simulink model "sampleModel167"  (R2021b)
settings: Solver=VariableStepAuto  StartTime=0.0  StopTime=10.0  RelTol=1e-3
undefined symbols (not defined in the file or in its folder): DiscIntNeverNeededParam
libraries: simulink x17, slpidlib x3, simulink_need_slupdate x2
settings Model: Creator=user  LastModifiedBy=user

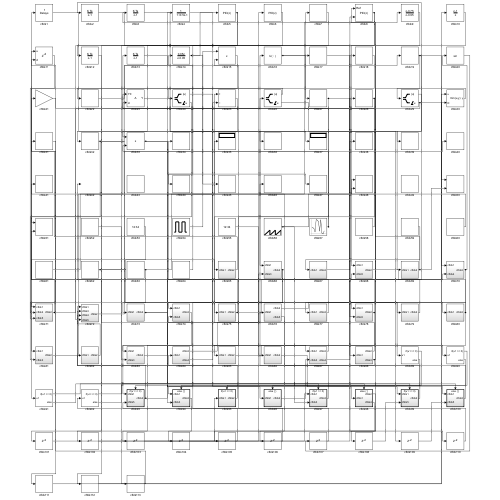
[thumbnail: Simulink's stored preview of the top-level diagram]
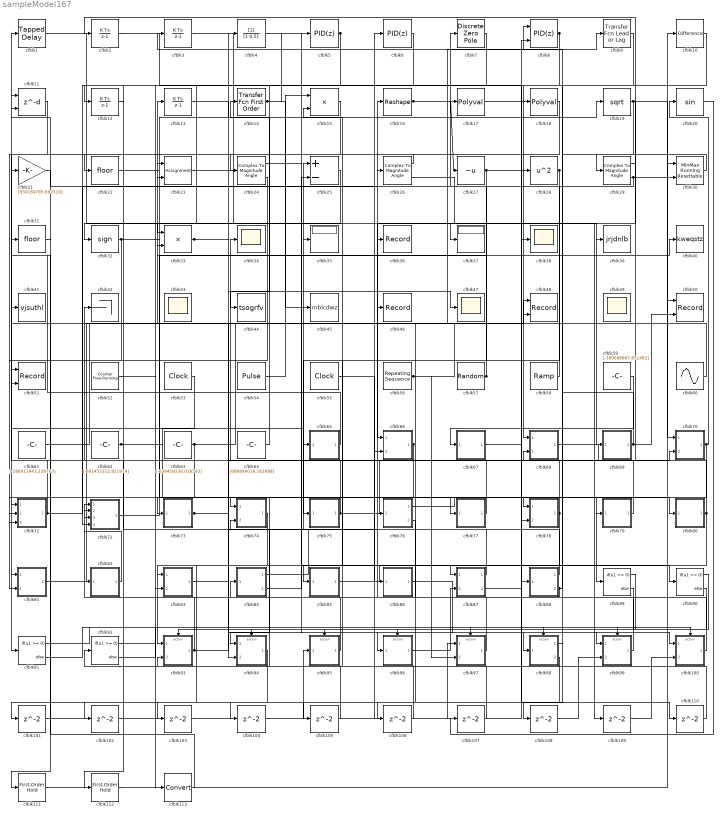
== system sampleModel167 ==
  cfblk1 : simulink/Discrete/Tapped Delay  vinit=0.0  samptime=-1  NumDelays=1  DelayOrder=Oldest  includeCurrent=off
  cfblk10 : simulink/Discrete/Difference  ICPrevInput=0.0  OutMin=[]  OutMax=[]  OutDataTypeStr=Inherit: Inherit via back propagation  OutDataType=fixdt(1, 16)  OutScaling=2^-10  DoSatur=off
  cfblk100 : Subsystem  TreatAsAtomicUnit=on
  cfblk{101..110} (10 alike) : Delay  SampleTime=1
  cfblk11 : Delay  DelayLengthSource=Input port  SampleTime=1
      settings: InputPortMap=u0,p1
  cfblk111 : simulink_need_slupdate/First-Order Hold  DisableCoverage=on  Ts=1
      settings: SourceProductBaseCode=SL
  cfblk112 : simulink_need_slupdate/First-Order Hold  DisableCoverage=on  Ts=1
      settings: SourceProductBaseCode=SL
  cfblk113 : DataTypeConversion
  cfblk{2..3,12..13} (4 alike) : DiscreteIntegrator  ICPrevOutput=DiscIntNeverNeededParam  ICPrevScaledInput=DiscIntNeverNeededParam
  cfblk14 : simulink/Discrete/Transfer Fcn First Order  PoleZ=0.95  ICPrevOutput=0.0  DoSatur=off
  cfblk15 : Product  Inputs=**
  cfblk16 : Reshape
  cfblk17 : Polyval  Coefs=[ +2.081618890e-019, -1.441693666e-014, +4.719686976e-010, -8.536869453e-006, +1.621573104e-001, -8.087801117e+001 ]
  cfblk18 : Polyval  Coefs=[ +2.081618890e-019, -1.441693666e-014, +4.719686976e-010, -8.536869453e-006, +1.621573104e-001, -8.087801117e+001 ]
  cfblk19 : Sqrt  SaturateOnIntegerOverflow=on
  cfblk20 : Trigonometry
  cfblk21 : Gain  Gain=[950169785.692510]
  cfblk22 : Rounding
  cfblk23 : Assignment  DiagnosticForDimensions=Warning  IndexOptions=Index vector (dialog)  Indices=1  OutputSizes=1
  cfblk24 : ComplexToMagnitudeAngle
  cfblk25 : Sum  Inputs=+-
  cfblk26 : ComplexToMagnitudeAngle
  cfblk27 : UnaryMinus
  cfblk28 : Math  Operator=square  SaturateOnIntegerOverflow=on
  cfblk29 : ComplexToMagnitudeAngle
  cfblk30 : simulink/Math Operations/MinMax Running Resettable  Function=min  vinit=0.0
  cfblk31 : Rounding
  cfblk32 : Signum
  cfblk33 : Product  Inputs=**
  cfblk{34,38,43,47,49} (5 alike) : Scope
      cfblk43 settings: Floating=on
      cfblk49 settings: Floating=on
  cfblk35 : Display
  cfblk36 : Record  FileSettingsInternal="{\"entries\":[{\"content\":{\"excelSettings\":{\"content\":{},\"type\":\"Streamout.ExcelSettings\"}},\"type\":\"Streamout.FileSettingStorage\",\"uuid\":\"ec53506d-30ea-4261-b9a0-b75c484f34c6\"}],\"packageUris\":[\"http://schema.mathworks.com/mf0/streamout_blocks/R2020a\"],\"version\":\"1.0\"}"  SignalsInternal="{\"entries\":[{\"content\":{\"signals\":[{\"content\":{\"blockPath\":[\"sampleModel167/cfblk36\"],\"channel\":[],\"dimensions\":[1],\"domain\":\"sampleModel167/cfblk36\",\"lineColor\":\"#0072bd\",\"plots\":[1],\"port\":1,\"sid\":[\"\"],\"signalID\":6249,\"signalName\":\"cfblk29:1\"},\"type\":\"RecordBlkView.Signal\",\"uuid\":\"139c6468-dbd3-450a-91ea-6cefff8656e1\"}]},\"type\":\"RecordBlkView.InputSignals\",\"uuid\":\"052d45fd-bfd9-46ee-adba-506bddab66a6\"}],\"packageUris\":[\"http://schema.mathworks.com/mf0/streamout_blocks/R2020a\"],\"version\":\"1.0\"}"  VisualizationBindings="{\"sparklinesplugin\":{\"info\":[{\"bindingParametersList\":[],\"subplotID\":1}]}}"
  cfblk37 : Display
  cfblk39 : ToWorkspace  VariableName=jrjdnlb  SaveFormat=Timeseries  SampleTime=-1
  cfblk4 : DiscreteFilter  SampleTime=1
  cfblk40 : ToWorkspace  VariableName=kweqstz  SaveFormat=Timeseries  SampleTime=-1
  cfblk41 : ToWorkspace  VariableName=vjsuthl  SaveFormat=Timeseries  SampleTime=-1
  cfblk42 : Terminator
  cfblk44 : ToWorkspace  VariableName=tsogrfv  SaveFormat=Timeseries  SampleTime=-1
  cfblk45 : ToWorkspace  VariableName=mblcdwz  SaveFormat=Timeseries  SampleTime=-1
  cfblk46 : Record  FileSettingsInternal="{\"entries\":[{\"content\":{\"excelSettings\":{\"content\":{},\"type\":\"Streamout.ExcelSettings\"}},\"type\":\"Streamout.FileSettingStorage\",\"uuid\":\"da6e1204-091f-4c4c-badc-bc2d25b8ce37\"}],\"packageUris\":[\"http://schema.mathworks.com/mf0/streamout_blocks/R2020a\"],\"version\":\"1.0\"}"  SignalsInternal="{\"entries\":[{\"content\":{\"signals\":[{\"content\":{\"blockPath\":[\"sampleModel167/cfblk46\"],\"channel\":[],\"dimensions\":[1],\"domain\":\"sampleModel167/cfblk46\",\"lineColor\":\"#d95319\",\"plots\":[1],\"port\":1,\"sid\":[\"\"],\"signalID\":6253,\"signalName\":\"cfblk100\"},\"type\":\"RecordBlkView.Signal\",\"uuid\":\"8a354596-a8b4-422e-ad70-63d130796eff\"}]},\"type\":\"RecordBlkView.InputSignals\",\"uuid\":\"d4f8df1c-8773-4cbd-9373-b1e680f83dd1\"}],\"packageUris\":[\"http://schema.mathworks.com/mf0/streamout_blocks/R2020a\"],\"version\":\"1.0\"}"  VisualizationBindings="{\"sparklinesplugin\":{\"info\":[{\"bindingParametersList\":[],\"subplotID\":1}]}}"
  cfblk48 : Record  FileSettingsInternal="{\"entries\":[{\"content\":{\"excelSettings\":{\"content\":{},\"type\":\"Streamout.ExcelSettings\"}},\"type\":\"Streamout.FileSettingStorage\",\"uuid\":\"2d2570bb-5f7a-4484-a74c-e022182345ca\"}],\"packageUris\":[\"http://schema.mathworks.com/mf0/streamout_blocks/R2020a\"],\"version\":\"1.0\"}"  Layout=[1 1]  SignalsInternal="{\"entries\":[{\"content\":{\"signals\":[{\"content\":{\"blockPath\":[\"sampleModel167/cfblk48\"],\"channel\":[],\"dimensions\":[1],\"domain\":\"sampleModel167/cfblk48\",\"lineColor\":\"#a2142f\",\"plots\":[1],\"port\":1,\"sid\":[\"\"],\"signalID\":6257,\"signalName\":\"cfblk80\"},\"type\":\"RecordBlkView.Signal\",\"uuid\":\"0f420bdd-d17e-44a9-89a2-4def85ddcdf1\"},{\"content\":{\"blockPath\":[\"sampleModel167/cfblk48\"],\"channel\":[],\"dimensions\":[1],\"domain\":\"sampleModel167/cfblk48\",\"lineColor\":\"#139fff\",\"plots\":[1],\"port\":2,\"sid\":[\"\"],\"signalID\":6261,\"signalName\":\"cfblk73\"},\"type\":\"RecordBlkView.Signal\",\"uuid\":\"37ea3ef6-358e-4351-b671-b7f0163bc937\"}]},\"type\":\"RecordBlkView.InputSignals\",\"uuid\":\"119d5875-aaf2-4c77-af19-f5638ded1561\"}],\"packageUris\":[\"http://schema.mathworks.com/mf0/streamout_blocks/R2020a\"],\"version\":\"1.0\"}"  VisualizationBindings="{\"xyplotplugin\":{\"info\":[{\"series\":[{\"bindingParametersList\":[{\"parameter\":\"X-Axis\",\"signalID\":6257,\"signalName\":\"cfblk80\"},{\"parameter\":\"Y-Axis\",\"signalID\":6261,\"signalName\":\"cfblk73\"}],\"seriesID\":53970}],\"subplotID\":1}]}}"  CompatibilityTag=XY
  cfblk5 : slpidlib/PID Controller  Controller=PID  Form=Parallel  TimeDomain=Discrete-time  UseExternalTs=off  SampleTime=1  IntegratorMethod=Forward Euler  FilterMethod=Forward Euler  ControllerParametersSource=internal  P=1  I=1  D=0  UseFilter=on  N=100  TunerSelectOption=Transfer Function Based (PID Tuner App)  InitialConditionSource=internal  InitialConditionForIntegrator=0  InitialConditionForFilter=0  DifferentiatorICPrevScaledInput=0  ExternalReset=none  TrackingMode=off  Kt=1  LimitOutput=off  SatLimitsSource=internal  UpperSaturationLimit=inf  LowerSaturationLimit=-inf  LinearizeAsGain=off  AntiWindupMode=none  Kb=1  POutMin=[]  POutMax=[]  IOutMin=[]  IOutMax=[]  DOutMin=[]  DOutMax=[]  NOutMin=[]  NOutMax=[]  SumOutMin=[]  SumOutMax=[]  SaturationOutMin=[]  SaturationOutMax=[]  PParamMin=[]  PParamMax=[]  IParamMin=[]  IParamMax=[]  DParamMin=[]  DParamMax=[]  NParamMin=[]  NParamMax=[]  KbParamMin=[]  KbParamMax=[]  KtParamMin=[]  KtParamMax=[]  KbOutMin=[]  KbOutMax=[]  KtOutMin=[]  KtOutMax=[]  IntegratorOutMin=[]  IntegratorOutMax=[]  FilterOutMin=[]  FilterOutMax=[]  SumI1OutMin=[]  SumI1OutMax=[]  SumI2OutMin=[]  SumI2OutMax=[]  SumI3OutMin=[]  SumI3OutMax=[]  SumI4OutMin=[]  SumI4OutMax=[]  SumDOutMin=[]  SumDOutMax=[]  DifferentiatorOutMin=[]  DifferentiatorOutMax=[]  FilterDiffOutCoefMin=[]  FilterDiffOutCoefMax=[]  ReciprocalOutMin=[]  ReciprocalOutMax=[]  SumDenOutMin=[]  SumDenOutMax=[]  SumNumOutMin=[]  SumNumOutMax=[]  DivideOutMin=[]  DivideOutMax=[]  UdiffTsProdOutMin=[]  UdiffTsProdOutMax=[]  NTsProdOutMin=[]  NTsProdOutMax=[]  UintegralTsProdOutMin=[]  UintegralTsProdOutMax=[]  UngainTsProdOutMin=[]  UngainTsProdOutMax=[]  IntegratorContinuousStateAttributes=''  IntegratorStateMustResolveToSignalObject=off  IntegratorRTWStateStorageClass=Auto  FilterContinuousStateAttributes=''  FilterStateMustResolveToSignalObject=off  FilterRTWStateStorageClass=Auto  ParallelPVariant=InternalParameters  IdealPVariant=Disabled  IVariant=InternalParameters  DVariant=InternalParameters  IntegratorVariant=Discrete  SatVariant=Disabled  AWVariant=Passthrough  PCopyVariant=Disabled  TRVariant=Disabled  FdbkBlocksVariant=Forward  IdealPFdbkVariant=Disabled  SatFdbkVariant=Disabled  DerivativeFilterVariant=ForwardEulerFilter  NVariant=InternalParameters  NCopyVariant=Disabled  FilterICVariant=InternalICsFilter  IntegratorICVariant=InternalICs  ExternalResetVariant=Disabled  TRSumVariant=Passthrough  SumFdbkVariant=Disabled  SumVariant=Sum_PID  TsampFilterVariant=InternalTs  TsampNgainVariant=Passthrough  TsampIntegralVariant=Passthrough  ExternalSaturationOutDataTypeStr=Inherit: Same as second input
  cfblk50 : Record  FileSettingsInternal="{\"entries\":[{\"content\":{\"excelSettings\":{\"content\":{},\"type\":\"Streamout.ExcelSettings\"}},\"type\":\"Streamout.FileSettingStorage\",\"uuid\":\"40a77355-b6b9-4623-865c-1ca23200a22d\"}],\"packageUris\":[\"http://schema.mathworks.com/mf0/streamout_blocks/R2020a\"],\"version\":\"1.0\"}"  Layout=[1 1]  SignalsInternal="{\"entries\":[{\"content\":{\"signals\":[{\"content\":{\"blockPath\":[\"sampleModel167/cfblk50\"],\"channel\":[],\"dimensions\":[1],\"domain\":\"sampleModel167/cfblk50\",\"lineColor\":\"#a2142f\",\"plots\":[1],\"port\":1,\"sid\":[\"\"],\"signalID\":6265,\"signalName\":\"cfblk29:2\"},\"type\":\"RecordBlkView.Signal\",\"uuid\":\"cc7a997b-e63d-444a-905f-d59d5b2896fd\"},{\"content\":{\"blockPath\":[\"sampleModel167/cfblk50\"],\"channel\":[],\"dimensions\":[1],\"domain\":\"sampleModel167/cfblk50\",\"lineColor\":\"#139fff\",\"plots\":[1],\"port\":2,\"sid\":[\"\"],\"signalID\":6269,\"signalName\":\"cfblk69\"},\"type\":\"RecordBlkView.Signal\",\"uuid\":\"124d10ed-abfe-4519-b392-b2a6d6e38794\"}]},\"type\":\"RecordBlkView.InputSignals\",\"uuid\":\"67c040a3-84bd-4415-84fd-296e2aa30a4d\"}],\"packageUris\":[\"http://schema.mathworks.com/mf0/streamout_blocks/R2020a\"],\"version\":\"1.0\"}"  VisualizationBindings="{\"xyplotplugin\":{\"info\":[{\"series\":[{\"bindingParametersList\":[{\"parameter\":\"X-Axis\",\"signalID\":6265,\"signalName\":\"cfblk29:2\"},{\"parameter\":\"Y-Axis\",\"signalID\":6269,\"signalName\":\"cfblk69\"}],\"seriesID\":27313}],\"subplotID\":1}]}}"  CompatibilityTag=XY
  cfblk51 : Record  FileSettingsInternal="{\"entries\":[{\"content\":{\"excelSettings\":{\"content\":{},\"type\":\"Streamout.ExcelSettings\"}},\"type\":\"Streamout.FileSettingStorage\",\"uuid\":\"e3204bcf-3174-4af1-beb2-6810d04cfba5\"}],\"packageUris\":[\"http://schema.mathworks.com/mf0/streamout_blocks/R2020a\"],\"version\":\"1.0\"}"  Layout=[1 1]  SignalsInternal="{\"entries\":[{\"content\":{\"signals\":[{\"content\":{\"blockPath\":[\"sampleModel167/cfblk51\"],\"channel\":[],\"dimensions\":[1],\"domain\":\"sampleModel167/cfblk51\",\"lineColor\":\"#a2142f\",\"plots\":[1],\"port\":1,\"sid\":[\"\"],\"signalID\":6273,\"signalName\":\"cfblk24:2\"},\"type\":\"RecordBlkView.Signal\",\"uuid\":\"6600f92a-317f-4508-8dc5-cdf654def4ef\"},{\"content\":{\"blockPath\":[\"sampleModel167/cfblk51\"],\"channel\":[],\"dimensions\":[1],\"domain\":\"sampleModel167/cfblk51\",\"lineColor\":\"#139fff\",\"plots\":[1],\"port\":2,\"sid\":[\"\"],\"signalID\":6277,\"signalName\":\"cfblk71\"},\"type\":\"RecordBlkView.Signal\",\"uuid\":\"6d6ba4b2-e462-4f03-bdb0-15236c8ce066\"}]},\"type\":\"RecordBlkView.InputSignals\",\"uuid\":\"fb1d1275-7641-4af6-b3e0-80677102a4a7\"}],\"packageUris\":[\"http://schema.mathworks.com/mf0/streamout_blocks/R2020a\"],\"version\":\"1.0\"}"  VisualizationBindings="{\"xyplotplugin\":{\"info\":[{\"series\":[{\"bindingParametersList\":[{\"parameter\":\"X-Axis\",\"signalID\":6273,\"signalName\":\"cfblk24:2\"},{\"parameter\":\"Y-Axis\",\"signalID\":6277,\"signalName\":\"cfblk71\"}],\"seriesID\":11353}],\"subplotID\":1}]}}"  CompatibilityTag=XY
  cfblk52 : simulink/Sources/Counter Free-Running  NumBits=[41.000000]  tsamp=-1
  cfblk53 : DigitalClock
  cfblk54 : DiscretePulseGenerator  PulseType=Time based  Amplitude=[534137876.527184]  Period=[54976083.843764]  PulseWidth=5  PhaseDelay=[8.000000]
  cfblk55 : DigitalClock
  cfblk56 : simulink/Sources/Repeating Sequence  rep_seq_t=[0 2]  rep_seq_y=[-841539136.031872, -579381442.323745]
  cfblk57 : RandomNumber  Mean=[-51850.961878]  Variance=[97939.194317]  Seed=[432152080.000000]  SampleTime=0.1
  cfblk58 : simulink/Sources/Ramp  slope=[-4478.791088]  start=[26.895940]  InitialOutput=[-682797.916035]
  cfblk59 : Constant  Value=[-369688867.851482]  SampleTime=1
  cfblk6 : slpidlib/PID Controller  Controller=PID  Form=Parallel  TimeDomain=Discrete-time  UseExternalTs=off  SampleTime=1  IntegratorMethod=Forward Euler  FilterMethod=Forward Euler  ControllerParametersSource=internal  P=1  I=1  D=0  UseFilter=on  N=100  TunerSelectOption=Transfer Function Based (PID Tuner App)  InitialConditionSource=internal  InitialConditionForIntegrator=0  InitialConditionForFilter=0  DifferentiatorICPrevScaledInput=0  ExternalReset=none  TrackingMode=off  Kt=1  LimitOutput=off  SatLimitsSource=internal  UpperSaturationLimit=inf  LowerSaturationLimit=-inf  LinearizeAsGain=off  AntiWindupMode=none  Kb=1  POutMin=[]  POutMax=[]  IOutMin=[]  IOutMax=[]  DOutMin=[]  DOutMax=[]  NOutMin=[]  NOutMax=[]  SumOutMin=[]  SumOutMax=[]  SaturationOutMin=[]  SaturationOutMax=[]  PParamMin=[]  PParamMax=[]  IParamMin=[]  IParamMax=[]  DParamMin=[]  DParamMax=[]  NParamMin=[]  NParamMax=[]  KbParamMin=[]  KbParamMax=[]  KtParamMin=[]  KtParamMax=[]  KbOutMin=[]  KbOutMax=[]  KtOutMin=[]  KtOutMax=[]  IntegratorOutMin=[]  IntegratorOutMax=[]  FilterOutMin=[]  FilterOutMax=[]  SumI1OutMin=[]  SumI1OutMax=[]  SumI2OutMin=[]  SumI2OutMax=[]  SumI3OutMin=[]  SumI3OutMax=[]  SumI4OutMin=[]  SumI4OutMax=[]  SumDOutMin=[]  SumDOutMax=[]  DifferentiatorOutMin=[]  DifferentiatorOutMax=[]  FilterDiffOutCoefMin=[]  FilterDiffOutCoefMax=[]  ReciprocalOutMin=[]  ReciprocalOutMax=[]  SumDenOutMin=[]  SumDenOutMax=[]  SumNumOutMin=[]  SumNumOutMax=[]  DivideOutMin=[]  DivideOutMax=[]  UdiffTsProdOutMin=[]  UdiffTsProdOutMax=[]  NTsProdOutMin=[]  NTsProdOutMax=[]  UintegralTsProdOutMin=[]  UintegralTsProdOutMax=[]  UngainTsProdOutMin=[]  UngainTsProdOutMax=[]  IntegratorContinuousStateAttributes=''  IntegratorStateMustResolveToSignalObject=off  IntegratorRTWStateStorageClass=Auto  FilterContinuousStateAttributes=''  FilterStateMustResolveToSignalObject=off  FilterRTWStateStorageClass=Auto  ParallelPVariant=InternalParameters  IdealPVariant=Disabled  IVariant=InternalParameters  DVariant=InternalParameters  IntegratorVariant=Discrete  SatVariant=Disabled  AWVariant=Passthrough  PCopyVariant=Disabled  TRVariant=Disabled  FdbkBlocksVariant=Forward  IdealPFdbkVariant=Disabled  SatFdbkVariant=Disabled  DerivativeFilterVariant=ForwardEulerFilter  NVariant=InternalParameters  NCopyVariant=Disabled  FilterICVariant=InternalICsFilter  IntegratorICVariant=InternalICs  ExternalResetVariant=Disabled  TRSumVariant=Passthrough  SumFdbkVariant=Disabled  SumVariant=Sum_PID  TsampFilterVariant=InternalTs  TsampNgainVariant=Passthrough  TsampIntegralVariant=Passthrough  ExternalSaturationOutDataTypeStr=Inherit: Same as second input
  cfblk60 : Sin  Amplitude=[-473951708.743377]  Bias=[-825559147.344328]  SampleTime=0
  cfblk61 : Constant  Value=[-188911943.228703]  SampleTime=1
  cfblk62 : Constant  Value=[-601452312.821979]  SampleTime=1
  cfblk63 : Constant  Value=[-638459236.016593]  SampleTime=1
  cfblk64 : Constant  Value=[686890016.162688]  SampleTime=1
  cfblk65 : Subsystem
  cfblk66 : Subsystem
  cfblk67 : Subsystem
  cfblk68 : Subsystem
  cfblk69 : Subsystem
  cfblk7 : DiscreteZeroPole  Poles=[0 0.5]  Gain=1
  cfblk70 : Subsystem
  cfblk71 : Subsystem
  cfblk72 : Subsystem
  cfblk73 : Subsystem
  cfblk74 : Subsystem
  cfblk75 : Subsystem
  cfblk76 : Subsystem
  cfblk77 : Subsystem
  cfblk78 : Subsystem
  cfblk79 : Subsystem
  cfblk8 : slpidlib/PID Controller (2DOF)  Controller=PID  Form=Parallel  TimeDomain=Discrete-time  UseExternalTs=off  SampleTime=1  IntegratorMethod=Forward Euler  FilterMethod=Forward Euler  ControllerParametersSource=internal  P=1  I=1  D=0  UseFilter=on  N=100  b=1  c=1  TunerSelectOption=Transfer Function Based (PID Tuner App)  InitialConditionSource=internal  InitialConditionForIntegrator=0  InitialConditionForFilter=0  DifferentiatorICPrevScaledInput=0  ExternalReset=none  TrackingMode=off  Kt=1  LimitOutput=off  SatLimitsSource=internal  UpperSaturationLimit=inf  LowerSaturationLimit=-inf  LinearizeAsGain=off  AntiWindupMode=none  Kb=1  POutMin=[]  POutMax=[]  IOutMin=[]  IOutMax=[]  DOutMin=[]  DOutMax=[]  NOutMin=[]  NOutMax=[]  bOutMin=[]  bOutMax=[]  cOutMin=[]  cOutMax=[]  SumOutMin=[]  SumOutMax=[]  SaturationOutMin=[]  SaturationOutMax=[]  PParamMin=[]  PParamMax=[]  IParamMin=[]  IParamMax=[]  DParamMin=[]  DParamMax=[]  NParamMin=[]  NParamMax=[]  bParamMin=[]  bParamMax=[]  cParamMin=[]  cParamMax=[]  KbParamMin=[]  KbParamMax=[]  KtParamMin=[]  KtParamMax=[]  KbOutMin=[]  KbOutMax=[]  KtOutMin=[]  KtOutMax=[]  IntegratorOutMin=[]  IntegratorOutMax=[]  FilterOutMin=[]  FilterOutMax=[]  SumI1OutMin=[]  SumI1OutMax=[]  SumI2OutMin=[]  SumI2OutMax=[]  SumI3OutMin=[]  SumI3OutMax=[]  SumI4OutMin=[]  SumI4OutMax=[]  SumDOutMin=[]  SumDOutMax=[]  Sum1OutMin=[]  Sum1OutMax=[]  Sum2OutMin=[]  Sum2OutMax=[]  Sum3OutMin=[]  Sum3OutMax=[]  DifferentiatorOutMin=[]  DifferentiatorOutMax=[]  FilterDiffOutCoefMin=[]  FilterDiffOutCoefMax=[]  ReciprocalOutMin=[]  ReciprocalOutMax=[]  SumDenOutMin=[]  SumDenOutMax=[]  SumNumOutMin=[]  SumNumOutMax=[]  DivideOutMin=[]  DivideOutMax=[]  UdiffTsProdOutMin=[]  UdiffTsProdOutMax=[]  NTsProdOutMin=[]  NTsProdOutMax=[]  UintegralTsProdOutMin=[]  UintegralTsProdOutMax=[]  UngainTsProdOutMin=[]  UngainTsProdOutMax=[]  IntegratorContinuousStateAttributes=''  IntegratorStateMustResolveToSignalObject=off  IntegratorRTWStateStorageClass=Auto  FilterContinuousStateAttributes=''  FilterStateMustResolveToSignalObject=off  FilterRTWStateStorageClass=Auto  ParallelPVariant=InternalParameters  IdealPVariant=Disabled  IVariant=InternalParameters  DVariant=InternalParameters  bVariant=InternalParameters  cVariant=InternalParameters  IntegratorVariant=Discrete  SatVariant=Disabled  AWVariant=Passthrough  PCopyVariant=Disabled  TRVariant=Disabled  FdbkBlocksVariant=Forward  IdealPFdbkVariant=Disabled  SatFdbkVariant=Disabled  DerivativeFilterVariant=ForwardEulerFilter  NVariant=InternalParameters  NCopyVariant=Disabled  FilterICVariant=InternalICsFilter  IntegratorICVariant=InternalICs  ExternalResetVariant=Disabled  TRSumVariant=Passthrough  SumFdbkVariant=Disabled  SumVariant=Sum_PID  TsampFilterVariant=InternalTs  TsampNgainVariant=Passthrough  TsampIntegralVariant=Passthrough  ExternalSaturationOutDataTypeStr=Inherit: Same as second input
      settings: SourceProductBaseCode=SL
  cfblk80 : Subsystem
  cfblk81 : Subsystem
  cfblk82 : Subsystem
  cfblk83 : Subsystem
  cfblk84 : Subsystem
  cfblk85 : Subsystem
  cfblk86 : Subsystem
  cfblk87 : Subsystem
  cfblk88 : Subsystem
  cfblk{89..92} (4 alike) : If  IfExpression=u1 >= 0  SampleTime=1
  cfblk9 : simulink/Discrete/Transfer Fcn Lead or Lag  PoleZ=0.95  ZeroZ=0.75  ICPrevOutput=0.0  ICPrevInput=0.0  DoSatur=off
      settings: SourceProductBaseCode=SL
  cfblk93 : Subsystem  TreatAsAtomicUnit=on
  cfblk94 : Subsystem  TreatAsAtomicUnit=on
  cfblk95 : Subsystem  TreatAsAtomicUnit=on
  cfblk96 : Subsystem  TreatAsAtomicUnit=on
  cfblk97 : Subsystem  TreatAsAtomicUnit=on
  cfblk98 : Subsystem  TreatAsAtomicUnit=on
  cfblk99 : Subsystem  TreatAsAtomicUnit=on
  wires:
  cfblk54/1 -> cfblk15/1
  cfblk25/1 -> cfblk32/1
  cfblk62/1 -> cfblk89/1, cfblk65/1(cfblk1)
  cfblk58/1 -> cfblk7/1
  cfblk16/1 -> cfblk27/1, cfblk9/1
  cfblk70/1(cfblk2) -> cfblk74/1(cfblk1), cfblk20/1
  cfblk88/1(cfblk2) -> cfblk1/1
  cfblk97/1(cfblk2) -> cfblk16/1
  cfblk69/1(cfblk2) -> cfblk8/1, cfblk50/2
  cfblk1/1 -> cfblk66/1(cfblk1)
  cfblk75/1(cfblk2) -> cfblk42/1, cfblk10/1
  cfblk61/1 -> cfblk13/1
  cfblk68/1(cfblk2) -> cfblk2/1
  cfblk79/1(cfblk2) -> cfblk11/1
  cfblk66/1(cfblk2) -> cfblk94/1(cfblk1), cfblk73/1(cfblk1)
  cfblk81/1(cfblk2) -> cfblk17/1
  cfblk11/1 -> cfblk91/1
  cfblk60/1 -> cfblk41/1
  cfblk77/1(cfblk2) -> cfblk34/1
  cfblk32/1 -> cfblk80/1(cfblk1), cfblk19/1, cfblk71/2(cfblk4)
  cfblk65/1(cfblk2) -> cfblk21/1
  cfblk59/1 -> cfblk67/1(cfblk1)
  cfblk14/1 -> cfblk5/1, cfblk45/1
  cfblk10/1 -> cfblk68/1(cfblk1)
  cfblk53/1 -> cfblk81/1(cfblk1)
  cfblk4/1 -> cfblk96/1(cfblk1)
  cfblk3/1 -> cfblk37/1
  cfblk13/1 -> cfblk94/2(cfblk3)
  cfblk93/1(cfblk2) -> cfblk72/1(cfblk1), cfblk76/1(cfblk1)
  cfblk6/1 -> cfblk12/1
  cfblk76/1(cfblk2) -> cfblk79/1(cfblk1)
  cfblk100/1(cfblk2) -> cfblk46/1
  cfblk71/1(cfblk2) -> cfblk26/1, cfblk51/2
  cfblk63/1 -> cfblk25/1, cfblk71/3(cfblk5)
  cfblk67/1(cfblk2) -> cfblk38/1
  cfblk21/1 -> cfblk71/1(cfblk1)
  cfblk74/1(cfblk2) -> cfblk93/1(cfblk1)
  cfblk86/1(cfblk2) -> cfblk98/1(cfblk1)
  cfblk57/1 -> cfblk11/2, cfblk33/2
  cfblk80/1(cfblk2) -> cfblk83/1(cfblk1), cfblk77/1(cfblk1), cfblk48/1
  cfblk29/1 -> cfblk36/1
  cfblk9/1 -> cfblk78/1(cfblk1)
  cfblk72/1(cfblk2) -> cfblk40/1
  cfblk78/1(cfblk2) -> cfblk68/2(cfblk5), cfblk103/1
  cfblk33/1 -> cfblk47/1, cfblk99/1(cfblk1)
  cfblk5/1 -> cfblk44/1, cfblk33/1
  cfblk73/1(cfblk2) -> cfblk100/1(cfblk1), cfblk48/2
  cfblk87/1(cfblk2) -> cfblk35/1
  cfblk23/1 -> cfblk69/1(cfblk1)
  cfblk85/1(cfblk2) -> cfblk90/1
  cfblk27/1 -> cfblk78/2(cfblk5), cfblk85/1(cfblk1)
  cfblk95/1(cfblk2) -> cfblk72/2(cfblk3)
  cfblk56/1 -> cfblk28/1, cfblk97/2(cfblk3)
  cfblk19/1 -> cfblk70/1(cfblk1), cfblk39/1, cfblk108/1
  cfblk55/1 -> cfblk86/1(cfblk1)
  cfblk24/1 -> cfblk87/1(cfblk1)
  cfblk28/1 -> cfblk75/1(cfblk1), cfblk23/2
  cfblk64/1 -> cfblk14/1
  cfblk15/1 -> cfblk81/2(cfblk3)
  cfblk22/1 -> cfblk4/1
  cfblk84/1(cfblk2) -> cfblk6/1
  cfblk2/1 -> cfblk88/1(cfblk1)
  cfblk99/1(cfblk2) -> cfblk84/1(cfblk1)
  cfblk96/1(cfblk2) -> cfblk87/2(cfblk3)
  cfblk26/1 -> cfblk24/1
  cfblk83/1(cfblk2) -> cfblk70/2(cfblk4)
  cfblk24/2 -> cfblk51/1
  cfblk84/2(cfblk4) -> cfblk25/2
  cfblk87/2(cfblk4) -> cfblk18/1
  cfblk7/1 -> cfblk22/1
  cfblk88/2(cfblk3) -> cfblk82/1(cfblk1), cfblk3/1
  cfblk29/2 -> cfblk50/1, cfblk23/1
  cfblk30/1 -> cfblk29/1
  cfblk8/1 -> cfblk83/2(cfblk3), cfblk72/4(cfblk5)
  cfblk82/1(cfblk2) -> cfblk72/3(cfblk4)
  cfblk89/1 -> cfblk93/Action
  cfblk89/2 -> cfblk94/Action
  cfblk90/1 -> cfblk95/Action
  cfblk90/2 -> cfblk96/Action
  cfblk91/1 -> cfblk97/Action
  cfblk91/2 -> cfblk98/Action
  cfblk92/1 -> cfblk99/Action
  cfblk92/2 -> cfblk100/Action
  cfblk94/1(cfblk2) -> cfblk101/1
  cfblk101/1 -> cfblk66/2(cfblk3)
  cfblk18/1 -> cfblk102/1
  cfblk102/1 -> cfblk95/1(cfblk1)
  cfblk103/1 -> cfblk97/1(cfblk1)
  cfblk98/1(cfblk2) -> cfblk104/1
  cfblk104/1 -> cfblk8/2
  cfblk98/2(cfblk4) -> cfblk105/1
  cfblk105/1 -> cfblk93/2(cfblk5)
  cfblk76/2(cfblk5) -> cfblk106/1
  cfblk106/1 -> cfblk74/2(cfblk5)
  cfblk20/1 -> cfblk107/1
  cfblk107/1 -> cfblk92/1
  cfblk108/1 -> cfblk99/2(cfblk5)
  cfblk26/2 -> cfblk109/1
  cfblk109/1 -> cfblk100/2(cfblk5)
  cfblk17/1 -> cfblk110/1
  cfblk110/1 -> cfblk15/2
  cfblk31/1 -> cfblk111/1
  cfblk111/1 -> cfblk30/1
  cfblk12/1 -> cfblk112/1
  cfblk112/1 -> cfblk30/2
  cfblk52/1 -> cfblk113/1
  cfblk113/1 -> cfblk31/1

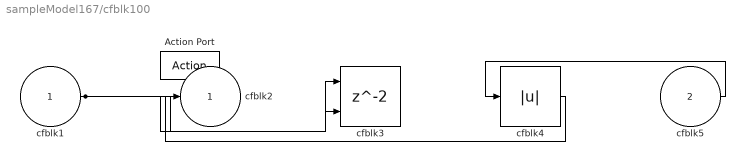
== system sampleModel167/cfblk100 ==
  cfblk1 : Inport
  cfblk5 : Inport  Port=2
  Action Port : ActionPort  ActionPortLabel=else
  cfblk3 : Delay  ShowEnablePort=on
      settings: InputPortMap=u0,e6
  cfblk4 : Abs
  cfblk2 : Outport
  wires:
  cfblk5/1 -> cfblk4/1
  cfblk1/1 -> cfblk3/1, cfblk3/2
  cfblk4/1 -> cfblk2/1

== system sampleModel167/cfblk65 ==
  cfblk1 : Inport
  cfblk3 : Sin  TimeSource=Use external signal  SampleTime=0
  cfblk4 : Constant  Value=[688240254.247042]  SampleTime=1
  cfblk2 : Outport
  wires:
  cfblk1/1 -> cfblk2/1
  cfblk4/1 -> cfblk3/1

== system sampleModel167/cfblk66 ==
  cfblk1 : Inport
  cfblk3 : Inport  Port=2
  cfblk2 : Outport
  wires:
  cfblk1/1 -> cfblk2/1

== system sampleModel167/cfblk67 ==
  cfblk1 : Inport
  cfblk3 : Constant  Value=[170733425.297575]  SampleTime=1
  cfblk2 : Outport
  wires:
  cfblk3/1 -> cfblk2/1

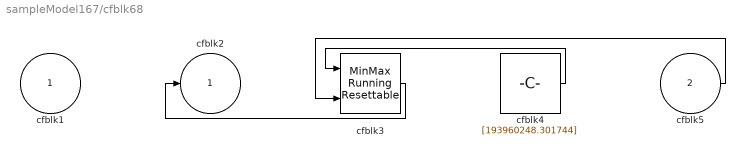
== system sampleModel167/cfblk68 ==
  cfblk1 : Inport
  cfblk5 : Inport  Port=2
  cfblk3 : simulink/Math Operations/MinMax Running Resettable  Function=min  vinit=0.0
  cfblk4 : Constant  Value=[193960248.301744]  SampleTime=1
  cfblk2 : Outport
  wires:
  cfblk4/1 -> cfblk3/1
  cfblk3/1 -> cfblk2/1
  cfblk5/1 -> cfblk3/2

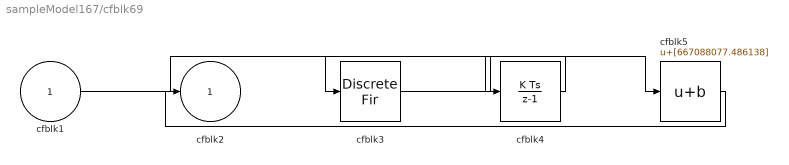
== system sampleModel167/cfblk69 ==
  cfblk1 : Inport
  cfblk3 : DiscreteFir  SampleTime=1
  cfblk4 : DiscreteIntegrator  ICPrevOutput=DiscIntNeverNeededParam  ICPrevScaledInput=DiscIntNeverNeededParam
  cfblk5 : Bias  Bias=[667088077.486138]
  cfblk2 : Outport
  wires:
  cfblk3/1 -> cfblk5/1
  cfblk1/1 -> cfblk4/1
  cfblk5/1 -> cfblk2/1
  cfblk4/1 -> cfblk3/1

== system sampleModel167/cfblk70 ==
  cfblk1 : Inport
  cfblk4 : Inport  Port=2
  cfblk3 : simulink/Discrete/Tapped Delay  vinit=0.0  samptime=-1  NumDelays=1  DelayOrder=Oldest  includeCurrent=off
  cfblk2 : Outport
  wires:
  cfblk1/1 -> cfblk2/1
  cfblk4/1 -> cfblk3/1

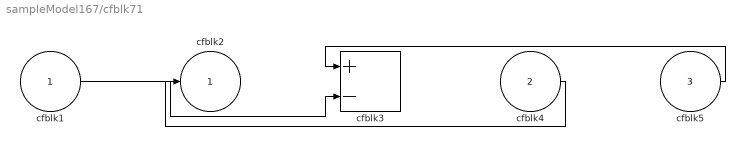
== system sampleModel167/cfblk71 ==
  cfblk1 : Inport
  cfblk4 : Inport  Port=2
  cfblk5 : Inport  Port=3
  cfblk3 : Sum  Inputs=+-
  cfblk2 : Outport
  wires:
  cfblk5/1 -> cfblk3/1
  cfblk1/1 -> cfblk3/2
  cfblk4/1 -> cfblk2/1

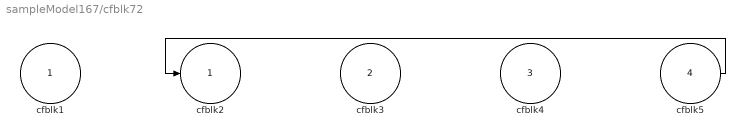
== system sampleModel167/cfblk72 ==
  cfblk1 : Inport
  cfblk3 : Inport  Port=2
  cfblk4 : Inport  Port=3
  cfblk5 : Inport  Port=4
  cfblk2 : Outport
  wires:
  cfblk5/1 -> cfblk2/1

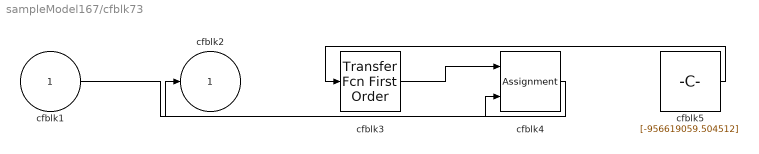
== system sampleModel167/cfblk73 ==
  cfblk1 : Inport
  cfblk3 : simulink/Discrete/Transfer Fcn First Order  PoleZ=0.95  ICPrevOutput=0.0  DoSatur=off
  cfblk4 : Assignment  DiagnosticForDimensions=Warning  IndexOptions=Index vector (dialog)  Indices=1  OutputSizes=1
  cfblk5 : Constant  Value=[-956619059.504512]  SampleTime=1
  cfblk2 : Outport
  wires:
  cfblk5/1 -> cfblk3/1
  cfblk3/1 -> cfblk4/1
  cfblk4/1 -> cfblk2/1
  cfblk1/1 -> cfblk4/2

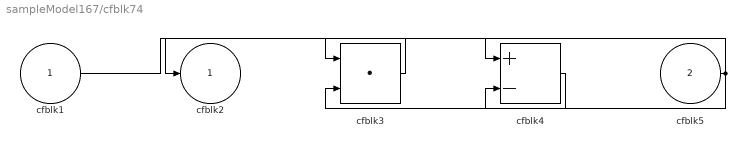
== system sampleModel167/cfblk74 ==
  cfblk1 : Inport
  cfblk5 : Inport  Port=2
  cfblk3 : DotProduct  InputSameDT=on  OutDataTypeStr=Inherit: Inherit via internal rule
  cfblk4 : Sum  Inputs=+-
  cfblk2 : Outport
  wires:
  cfblk5/1 -> cfblk3/1, cfblk4/2
  cfblk4/1 -> cfblk3/2
  cfblk3/1 -> cfblk2/1
  cfblk1/1 -> cfblk4/1

== system sampleModel167/cfblk75 ==
  cfblk1 : Inport
  cfblk3 : Trigonometry
  cfblk2 : Outport
  wires:
  cfblk3/1 -> cfblk2/1
  cfblk1/1 -> cfblk3/1

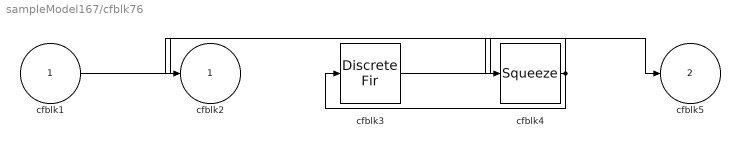
== system sampleModel167/cfblk76 ==
  cfblk1 : Inport
  cfblk3 : DiscreteFir  SampleTime=1
  cfblk4 : Squeeze
  cfblk2 : Outport
  cfblk5 : Outport  Port=2
  wires:
  cfblk3/1 -> cfblk5/1
  cfblk1/1 -> cfblk4/1
  cfblk4/1 -> cfblk3/1, cfblk2/1

== system sampleModel167/cfblk77 ==
  cfblk1 : Inport
  cfblk3 : DiscreteTransferFcn  SampleTime=1
  cfblk4 : Sum  Inputs=-+
  cfblk5 : simulink/Math Operations/Slider Gain  gain=1  low=0  high=2
  cfblk2 : Outport
  wires:
  cfblk1/1 -> cfblk3/1
  cfblk3/1 -> cfblk4/1, cfblk5/1
  cfblk4/1 -> cfblk2/1
  cfblk5/1 -> cfblk4/2

== system sampleModel167/cfblk78 ==
  cfblk1 : Inport
  cfblk5 : Inport  Port=2
  cfblk3 : DiscreteZeroPole  Poles=[0 0.5]  Gain=1
  cfblk4 : simulink/Discrete/Transfer Fcn Lead or Lag  PoleZ=0.95  ZeroZ=0.75  ICPrevOutput=0.0  ICPrevInput=0.0  DoSatur=off
      settings: SourceProductBaseCode=SL
  cfblk2 : Outport
  wires:
  cfblk5/1 -> cfblk3/1
  cfblk1/1 -> cfblk2/1
  cfblk3/1 -> cfblk4/1

== system sampleModel167/cfblk79 ==
  cfblk1 : Inport
  cfblk3 : simulink/Discrete/Difference  ICPrevInput=0.0  OutMin=[]  OutMax=[]  OutDataTypeStr=Inherit: Inherit via back propagation  OutDataType=fixdt(1, 16)  OutScaling=2^-10  DoSatur=off
  cfblk4 : Sqrt  SaturateOnIntegerOverflow=on
  cfblk2 : Outport
  wires:
  cfblk1/1 -> cfblk3/1, cfblk4/1
  cfblk3/1 -> cfblk2/1

== system sampleModel167/cfblk80 ==
  cfblk1 : Inport
  cfblk3 : Sum  Inputs=|++
  cfblk4 : Product
  cfblk5 : Delay  SampleTime=1
  cfblk2 : Outport
  wires:
  cfblk1/1 -> cfblk4/1, cfblk3/2
  cfblk4/1 -> cfblk2/1, cfblk3/1
  cfblk3/1 -> cfblk5/1
  cfblk5/1 -> cfblk4/2

== system sampleModel167/cfblk81 ==
  cfblk1 : Inport
  cfblk3 : Inport  Port=2
  cfblk2 : Outport
  wires:
  cfblk1/1 -> cfblk2/1

== system sampleModel167/cfblk82 ==
  cfblk1 : Inport
  cfblk3 : simulink/Discrete/Transfer Fcn First Order  PoleZ=0.95  ICPrevOutput=0.0  DoSatur=off
  cfblk4 : Rounding
  cfblk5 : Abs
  cfblk2 : Outport
  wires:
  cfblk1/1 -> cfblk3/1
  cfblk4/1 -> cfblk2/1
  cfblk3/1 -> cfblk5/1
  cfblk5/1 -> cfblk4/1

== system sampleModel167/cfblk83 ==
  cfblk1 : Inport
  cfblk3 : Inport  Port=2
  cfblk2 : Outport
  wires:
  cfblk3/1 -> cfblk2/1

== system sampleModel167/cfblk84 ==
  cfblk1 : Inport
  cfblk3 : Bias  Bias=[-785996035.115216]
  cfblk2 : Outport
  cfblk4 : Outport  Port=2
  wires:
  cfblk1/1 -> cfblk4/1, cfblk3/1
  cfblk3/1 -> cfblk2/1

== system sampleModel167/cfblk85 ==
  cfblk1 : Inport
  cfblk3 : DiscreteTransferFcn  SampleTime=1
  cfblk2 : Outport
  wires:
  cfblk1/1 -> cfblk2/1, cfblk3/1

== system sampleModel167/cfblk86 ==
  cfblk1 : Inport
  cfblk3 : simulink/Discrete/Transfer Fcn First Order  PoleZ=0.95  ICPrevOutput=0.0  DoSatur=off
  cfblk4 : Reshape
  cfblk2 : Outport
  wires:
  cfblk3/1 -> cfblk4/1
  cfblk1/1 -> cfblk3/1
  cfblk4/1 -> cfblk2/1

== system sampleModel167/cfblk87 ==
  cfblk1 : Inport
  cfblk3 : Inport  Port=2
  cfblk2 : Outport
  cfblk4 : Outport  Port=2
  wires:
  cfblk1/1 -> cfblk2/1
  cfblk3/1 -> cfblk4/1

== system sampleModel167/cfblk88 ==
  cfblk1 : Inport
  cfblk2 : Outport
  cfblk3 : Outport  Port=2
  wires:
  cfblk1/1 -> cfblk3/1, cfblk2/1

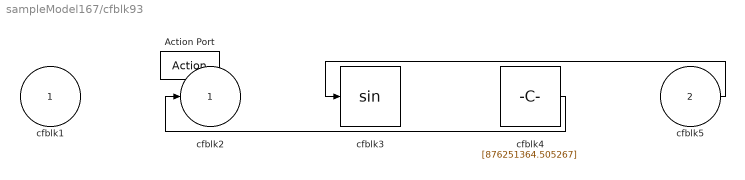
== system sampleModel167/cfblk93 ==
  cfblk1 : Inport
  cfblk5 : Inport  Port=2
  Action Port : ActionPort  ActionPortLabel=if(u1 >= 0)
  cfblk3 : Trigonometry
  cfblk4 : Constant  Value=[876251364.505267]  SampleTime=1
  cfblk2 : Outport
  wires:
  cfblk4/1 -> cfblk2/1
  cfblk5/1 -> cfblk3/1

== system sampleModel167/cfblk94 ==
  cfblk1 : Inport
  cfblk3 : Inport  Port=2
  Action Port : ActionPort  ActionPortLabel=else
  cfblk2 : Outport
  wires:
  cfblk3/1 -> cfblk2/1

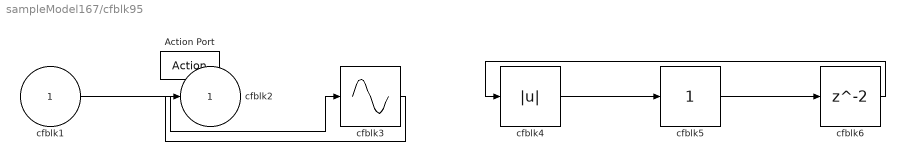
== system sampleModel167/cfblk95 ==
  cfblk1 : Inport
  Action Port : ActionPort  ActionPortLabel=if(u1 >= 0)
  cfblk3 : Sin  TimeSource=Use external signal  SampleTime=0
  cfblk4 : Abs
  cfblk5 : simulink/Math Operations/Slider Gain  gain=1  low=0  high=2
  cfblk6 : Delay
  cfblk2 : Outport
  wires:
  cfblk1/1 -> cfblk3/1
  cfblk4/1 -> cfblk5/1
  cfblk3/1 -> cfblk2/1
  cfblk5/1 -> cfblk6/1
  cfblk6/1 -> cfblk4/1

== system sampleModel167/cfblk96 ==
  cfblk1 : Inport
  Action Port : ActionPort  ActionPortLabel=else
  cfblk3 : Sum  Inputs=|++
  cfblk2 : Outport
  wires:
  cfblk1/1 -> cfblk3/1, cfblk3/2
  cfblk3/1 -> cfblk2/1

== system sampleModel167/cfblk97 ==
  cfblk1 : Inport
  cfblk3 : Inport  Port=2
  Action Port : ActionPort  ActionPortLabel=if(u1 >= 0)
  cfblk2 : Outport
  wires:
  cfblk1/1 -> cfblk2/1

== system sampleModel167/cfblk98 ==
  cfblk1 : Inport
  Action Port : ActionPort  ActionPortLabel=else
  cfblk3 : DiscreteFir
  cfblk2 : Outport
  cfblk4 : Outport  Port=2
  wires:
  cfblk1/1 -> cfblk2/1, cfblk3/1
  cfblk3/1 -> cfblk4/1

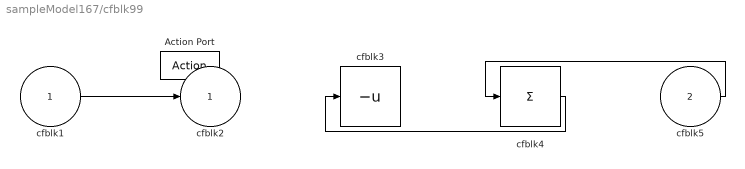
== system sampleModel167/cfblk99 ==
  cfblk1 : Inport
  cfblk5 : Inport  Port=2
  Action Port : ActionPort  ActionPortLabel=if(u1 >= 0)
  cfblk3 : UnaryMinus
  cfblk4 : Sum  Inputs=+
  cfblk2 : Outport
  wires:
  cfblk1/1 -> cfblk2/1
  cfblk5/1 -> cfblk4/1
  cfblk4/1 -> cfblk3/1
